simulink library "Resettable_Unit_Delay"  (R2020b)
settings: Solver=VariableStepAuto  StartTime=0.0  StopTime=10.0  RelTol=1e-3
undefined symbols (not defined in the file or in its folder): en_ResetStates, PauseResume
settings Model: Creator=matteolarcher  LastModifiedBy=matteolarcher

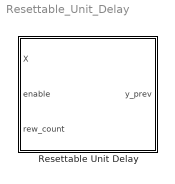
== system Resettable_Unit_Delay ==
  Resettable Unit Delay : Subsystem  mask{Ts_int=0.001, X0_int=0, en_res_flag=en_ResetStates}
      mask prompts: Ts_int "sampling time"; X0_int "initial conditions"; en_res_flag "enable_reset_flag"

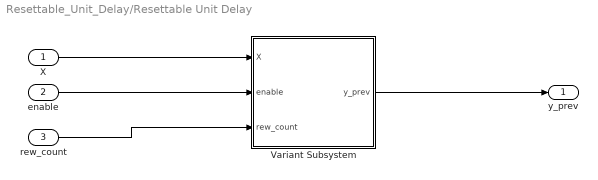
== system Resettable_Unit_Delay/Resettable Unit Delay ==
  X : Inport
  enable : Inport  Port=2
  rew_count : Inport  Port=3
  Variant Subsystem : Subsystem  Variant=on
  y_prev : Outport
  wires:
  X/1 -> Variant Subsystem/1(X)
  enable/1 -> Variant Subsystem/2(enable)
  rew_count/1 -> Variant Subsystem/3(rew_count)
  Variant Subsystem/1(y_prev) -> y_prev/1

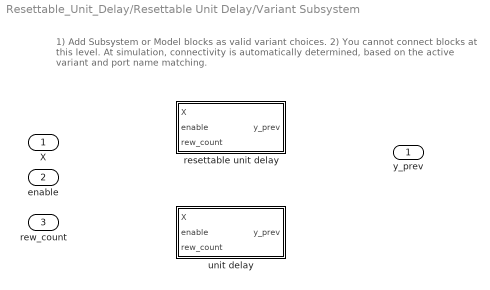
== system Resettable_Unit_Delay/Resettable Unit Delay/Variant Subsystem ==
  note: 1) Add Subsystem or Model blocks as valid variant choices.
      | 2) You cannot connect blocks at this level. At simulation, connectivity is automatically
      | determined, based on the active variant and port name matching.
  X : Inport
  enable : Inport  Port=2
  rew_count : Inport  Port=3
  resettable unit delay : Subsystem  VariantControl=en_res_flag == 1
  unit delay : Subsystem  VariantControl=en_res_flag == 0
  y_prev : Outport

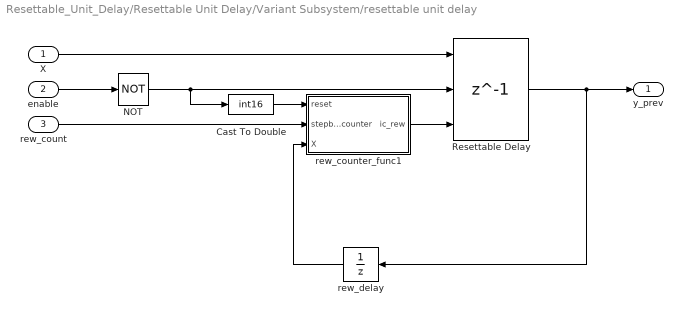
== system Resettable_Unit_Delay/Resettable Unit Delay/Variant Subsystem/resettable unit delay ==
  X : Inport
  enable : Inport  Port=2
  rew_count : Inport  Port=3
  Cast To Double : DataTypeConversion  OutDataTypeStr=int16
  NOT : Logic  Operator=NOT  IconShape=distinctive  AllPortsSameDT=off  OutDataTypeStr=boolean
  Resettable Delay : Delay  DelayLength=1  InitialConditionSource=Input port  ExternalReset=Level
      settings: InputPortMap=u0,r5,p4
  rew_counter_func1 : MATLAB Function  TreatAsAtomicUnit=on
  rew_delay : UnitDelay  SampleTime=Ts_int  HasFrameUpgradeWarning=on
  y_prev : Outport
  wires:
  rew_delay/1 -> rew_counter_func1/3(X)
  rew_counter_func1/1(ic_rew) -> Resettable Delay/3
  rew_count/1 -> rew_counter_func1/2(stepback_counter)
  enable/1 -> NOT/1
  Resettable Delay/1 -> y_prev/1, rew_delay/1
  X/1 -> Resettable Delay/1
  NOT/1 -> Cast To Double/1, Resettable Delay/2
  Cast To Double/1 -> rew_counter_func1/1(reset)

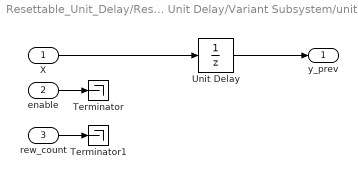
== system Resettable_Unit_Delay/Resettable Unit Delay/Variant Subsystem/unit delay ==
  X : Inport
  enable : Inport  Port=2
  rew_count : Inport  Port=3
  Terminator : Terminator
  Terminator1 : Terminator
  Unit Delay : UnitDelay  InitialCondition=X0_int  SampleTime=Ts_int  HasFrameUpgradeWarning=on
  y_prev : Outport
  wires:
  enable/1 -> Terminator/1
  rew_count/1 -> Terminator1/1
  X/1 -> Unit Delay/1
  Unit Delay/1 -> y_prev/1

== matlab function Resettable_Unit_Delay/Resettable Unit Delay/Variant Subsystem/resettable unit delay/rew_counter_func1 ==
  data: reset input; stepback_counter input; X input; ic_rew output; X0_int parameter; Ts_int parameter; PauseResume parameter
%% VEHICLE REWIND STATES

function ic_rew = ic_buffer(reset, stepback_counter, X, X0_int, Ts_int, PauseResume)

persistent states_buf i reset_pre

% safety saturations
if PauseResume.rewind_time > 50
    n_states = 50;
else
    n_states = PauseResume.rewind_time;
end
if stepback_counter > n_states
    stepback_counter = int16(n_states);
end

% initialization

size_fifo = size(X0_int,2);
ic_rew = zeros(1,size_fifo);
if isempty(states_buf)
    states_buf = zeros(int16(n_states), size_fifo);
    for j=1:n_states
        states_buf(j,:) = X;
    end
end
if isempty(i)
   i = 0;
end
if isempty(reset_pre)
   reset_pre = int16(0);
end

%%%%%%%%%%

% update buffer every rewind_samp 
if mod(i,PauseResume.rewind_samp/Ts_int)==0 && reset==0 && reset_pre==0
    states_buf(2:end,:) = states_buf(1:end-1,:);
    states_buf(1,:) = X;
end

% update initial conditions
if stepback_counter > 0     % stepback resume
    ic_rew(1,:) = states_buf(stepback_counter, :);
else                        % pause-resume without stepback 
    ic_rew(1,:) = X;
end

% detect enable falling edge and update buffer
% selected
if reset_pre > reset
    remain_size = n_states-stepback_counter+1;              % number of samples older than stepback_counter to be keep
    states_buf(1:remain_size, :) = states_buf(stepback_counter:end, :);    % porto in cima alla fifo i valori rimasti del buffer più vecchi di stepback_counter
    for j=remain_size+1:n_states
        states_buf(j, :) = states_buf(remain_size, :);         % riempio la fifo con l'ultimo valore buono 
    end 
end

% increase counter
i = i+1;
reset_pre = reset;
     
end
